simulink subsystem "ControllerBA"  (R2023b)
settings: Solver=VariableStepAuto  StartTime=0.0  StopTime=10.0  RelTol=1e-3
settings Model: Creator=juana  LastModifiedBy=juana

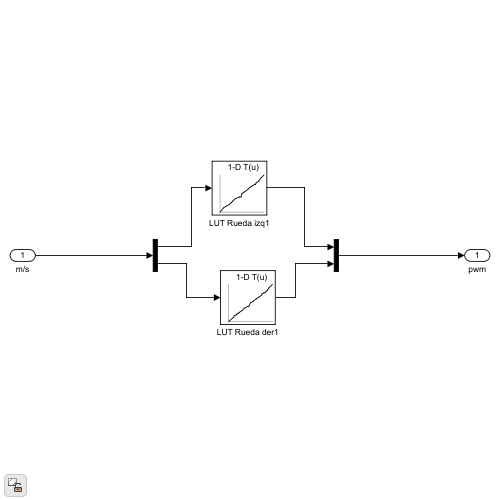
[thumbnail: Simulink's stored preview of the top-level diagram]
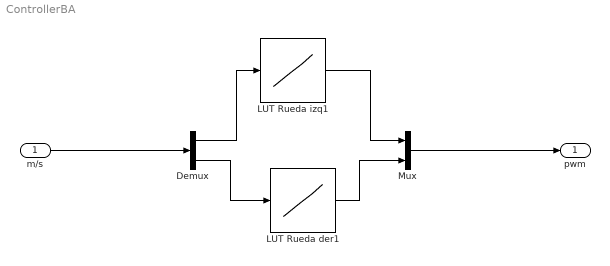
== system ControllerBA ==
  m/s : Inport
  Demux : Demux  Outputs=2
  LUT Rueda der1 : Lookup_n-D  NumberOfTableDimensions=1  BreakpointsForDimension1=[-0.665946960449219;-0.523246765136719;-0.475685119628906;-0.428115844726563;-0.404335021972656;-0.356758117675781;-0.332969665527344;-0.261619567871094;-0.190277099609375;-0.095123291015625;-0.0475616455078125;0;0.0713653564453125;0.166488647460938;0.23785400390625;0.309196472167969;0.356758117675781;0.404327392578125;0.451896667480469;0.499465942382813;0.547035217285156;0.642169952392578]  Table=[-254;-200.65998840332;-175.259948730469;-162.559967041016;-149.859985351563;-134.619995117188;-125.729972839355;-100.32999420166;-74.9299621582031;-50.8000106811523;-44.4499893188477;0;25.500036239624;51.0000114440918;75.2249908447266;100.724998474121;124.949989318848;135.150024414063;150.450012207031;174.674987792969;200.175018310547;255]  InternalRulePriority=Speed  RndMeth=Simplest
  LUT Rueda izq1 : Lookup_n-D  NumberOfTableDimensions=1  BreakpointsForDimension1=[-0.665946960449219;-0.547027587890625;-0.475677490234375;-0.380546569824219;-0.332977294921875;-0.285415649414063;-0.190277099609375;-0.07135009765625;-0.023773193359375;0;0.0713653564453125;0.190261840820313;0.237838745117188;0.309188842773438;0.380538940429688;0.404327392578125;0.451904296875;0.52325439453125;0.570823669433594;0.665946960449219]  Table=[-254;-200.65998840332;-175.259948730469;-149.859985351563;-125.729972839355;-100.32999420166;-74.9299621582031;-50.8000106811523;-44.4499893188477;0;25.500036239624;51.0000114440918;75.2249908447266;100.724998474121;124.949989318848;130.050003051758;150.450012207031;174.674987792969;200.175018310547;255]  InternalRulePriority=Speed  RndMeth=Simplest
  Mux : Mux  Inputs=2
  pwm : Outport
  wires:
  m/s/1 -> Demux/1
  Mux/1 -> pwm/1
  Demux/1 -> LUT Rueda izq1/1
  LUT Rueda izq1/1 -> Mux/1
  Demux/2 -> LUT Rueda der1/1
  LUT Rueda der1/1 -> Mux/2
